simulink model "gravitational_force"  (R2020b)
settings: Solver=FixedStepAuto  StartTime=0.0  StopTime=10.0  RelTol=1e-3
undefined symbols (not defined in the file): C_g, P_m_rocket
settings Model: Creator=Nicolai  LastModifiedBy=Nicolai

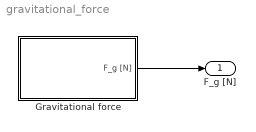
== system gravitational_force ==
  Gravitational force : Subsystem
  F_g [N] : Outport
  wires:
  Gravitational force/1(F_g [N]) -> F_g [N]/1

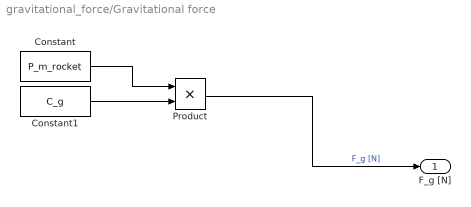
== system gravitational_force/Gravitational force ==
  Constant : Constant  Value=P_m_rocket
  Constant1 : Constant  Value=C_g
  Product : Product
  F_g [N] : Outport
  wires:
  Constant1/1 -> Product/2
  Constant/1 -> Product/1
  Product/1 -> F_g [N]/1  "F_g [N]"
